simulink library "dspspect3"  (Simulink 6.0)
undefined symbols (not defined in the file or in its folder): D, magnitude
libraries: dspspect3 x5, dspparest3 x4, dspsigattribs x2, dspsigops x2, dspxfrm3 x1, dsparch4 x1, simulink x1
settings Model: RequirementInfo=9  CovMetricSettings=d  ForwardingTableString=||__slOldName__||dspspect3/Short-Time FFT||__slNewName__||dspspect3/Periodogram  Creator=don  LastModifiedBy=sconahan  ExtModeAutoUpdateStatusClock=off  ProdHWDeviceType=Specified

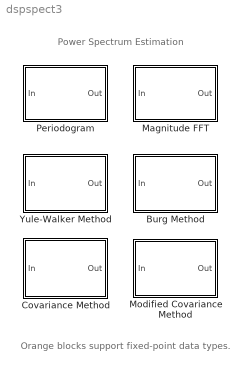
== system dspspect3 ==
  note: Power Spectrum Estimation
  note: Orange blocks support fixed-point data types.
  Burg Method : Subsystem  mask(Burg Method){inheritOrd=off, ord=6, inheritFFT=off, fftsize=256}
      mask prompts: inheritOrd "Inherit estimation order from input dimensions"; ord "Estimation order:"; inheritFFT "Inherit FFT length from estimation order"; fftsize "FFT length:"
      mask help: Parametric estimation of the AR spectrum using the Burg method.
      mask init:
      | [xe,x,y]=dspblkburgmeth2('icon');
      | dspblkburgmeth2('init');
      mask Help: web(dspbhelp);
      mask CallbackString: dspblkburgmeth2||dspblkburgmeth2|
      mask Display: text(-3,1.2,'Burg'); plot(-xe,0,xe,1.3,x,y)
  Covariance Method : Subsystem  mask(Covariance Method){ord=6, inheritFFT=off, fftsize=256}
      mask prompts: ord "Estimation order:"; inheritFFT "Inherit FFT length from estimation order"; fftsize "FFT length:"
      mask help: Parametric estimation of the AR spectrum using the covariance method.
      mask init:
      | [xe,x,y]=dspblkcovarmeth2('icon');
      | dspblkcovarmeth2('init');
      mask Help: web(dspbhelp);
      mask CallbackString: |dspblkcovarmeth2|
      mask Display: text(-3,1.2,'Cov AR'); plot(-xe,0,xe,1.3,x,y)
  Magnitude FFT : Subsystem  mask(Magnitude FFT){mag_or_magsq=Magnitude squared, fftLenInherit=off, fftsize=256}
      mask prompts: mag_or_magsq "Output:"; fftLenInherit "Inherit FFT length from input dimensions"; fftsize "FFT length:"
      mask help: Compute magnitude or magnitude-squared FFT of the input, with optional zero padding.
      mask init:
      | str=dspblkmagfft2('init');dspblkmagfft2('update');
      settings: CopyFcn=dspfixptcopycallback
      mask Help: web(dspbhelp);
      mask StyleString: popup(Magnitude squared|Magnitude),checkbox,edit
      mask CallbackString: |dspblkmagfft2;|
      mask Display: disp(str,'texmode','on');
  Modified Covariance Method : Subsystem  mask(Modified Covariance Method){ord=6, inheritFFT=off, fftsize=256}
      mask prompts: ord "Estimation order:"; inheritFFT "Inherit FFT length from estimation order"; fftsize "FFT length:"
      mask help: Parametric estimation of the AR spectrum using the modified covariance method.
      mask init:
      | [xe,x,y]=dspblkmodcovmeth2('icon');
      | dspblkmodcovmeth2('init');
      mask Help: web(dspbhelp);
      mask CallbackString: |dspblkmodcovmeth2|
      mask Display: text(-3,1.2,'MCov AR'); plot(-xe,0,xe,1.3,x,y)
  Periodogram : Subsystem  mask(Periodogram){wintype=Hamming, Rs=50, beta=5, winsamp=Symmetric, inheritFFT=off, fftsize=256, navg=4}
      mask prompts: wintype "Window type:"; Rs "Stopband attenuation in dB:"; winsamp "Window sampling:"; inheritFFT "Inherit FFT length from input dimensions"; fftsize "FFT length:"; navg "Number of spectral averages:"
      mask help: Nonparametric spectral estimation using the Periodogram method.
      mask init:
      | [x,y,xe]=dspblkshorttimefft2('icon');
      | dspblkshorttimefft2('init');
      mask Help: web(dspbhelp);
      mask StyleString: popup(Bartlett|Blackman|Boxcar|Chebyshev|Hamming|Hann|Hanning|Kaiser|Triang),edit,edit,popup(Symmetric|Periodic),checkbox,edit,edit
      mask CallbackString: dspblkshorttimefft2||||dspblkshorttimefft2||
      mask Display:
      | text(-3,1.15,'Periodogram');
      | plot((-xe),0,xe,1.3,x,y)
  Yule-Walker Method : Subsystem  mask(Yule-Walker Method){inheritOrd=off, ord=6, inheritFFT=off, fftsize=256}
      mask prompts: inheritOrd "Inherit estimation order from input dimensions"; ord "Estimation order:"; inheritFFT "Inherit FFT length from estimation order"; fftsize "FFT length:"
      mask help: Parametric estimation of the AR spectrum using the autocorrelation (LPC) method.
      mask init:
      | [xe,x,y]=dspblkyulewalkmeth2('icon');
      | dspblkyulewalkmeth2('init');
      mask Help: web(dspbhelp);
      mask CallbackString: dspblkyulewalkmeth2||dspblkyulewalkmeth2|
      mask Display: text(-3,1.2,'Yule AR'); plot(-xe,0,xe,1.3,x,y)

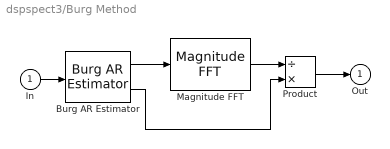
== system dspspect3/Burg Method ==
  In : Inport
  Burg AR Estimator : dspparest3/Burg AR Estimator  fcn=A  inheritOrder=off  ord=ord
  Magnitude FFT : dspspect3/Magnitude FFT  mag_or_magsq=Magnitude squared  fftLenInherit=off  fftsize=fftsize
  Product : Product  Inputs=/*  SaturateOnIntegerOverflow=on  InputSameDT=on
  Out : Outport  InitialOutput=0
  wires:
  In/1 -> Burg AR Estimator/1
  Burg AR Estimator/1 -> Magnitude FFT/1
  Magnitude FFT/1 -> Product/1
  Burg AR Estimator/2 -> Product/2
  Product/1 -> Out/1

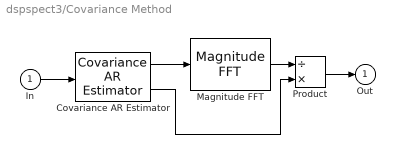
== system dspspect3/Covariance Method ==
  In : Inport
  Covariance AR Estimator : dspparest3/Covariance AR Estimator  P=ord
  Magnitude FFT : dspspect3/Magnitude FFT  mag_or_magsq=Magnitude squared  fftLenInherit=off  fftsize=fftsize
  Product : Product  Inputs=/*  SaturateOnIntegerOverflow=on  InputSameDT=on
  Out : Outport  InitialOutput=0
  wires:
  Magnitude FFT/1 -> Product/1
  Product/1 -> Out/1
  Covariance AR Estimator/1 -> Magnitude FFT/1
  Covariance AR Estimator/2 -> Product/2
  In/1 -> Covariance AR Estimator/1

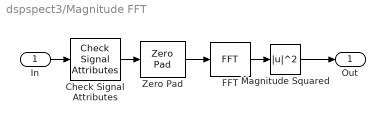
== system dspspect3/Magnitude FFT ==
  In : Inport
  Check Signal Attributes : dspsigattribs/Check Signal Attributes  SigAttribCheckMethod=Matches attributes exactly  Complexity=Ignore  Frame=Sample-based  DimsCheckMethod=Is...  Dimensions=Row vector (2-D)  DatatypeCheckMethod=Ignore  DatatypeGeneral=Boolean  DtypeFloatSpecific=Any floating-point  DtypeFixedSpecific=Any fixed-point  DtypeIntSpecific=Any integer  SampleMode=Ignore
  FFT : dspxfrm3/FFT  CompMethod=Table lookup  TableOpt=Speed  BitRevOrder=off  SkipNorm=on  roundingMode=Floor  overflowMode=off
  Magnitude Squared : Math  Operator=magnitude^2  ShowAdditionalParam=on  SaturateOnIntegerOverflow=on
  Zero Pad : dspsigops/Zero Pad  padSigAt=End  zpadAlong=Columns  padNumOutRowsSpecMethod=User-specified  numOutRows=fftsize  padNumOutColsSpecMethod=User-specified  numOutCols=1  trunc_flag=None
  Out : Outport
  wires:
  Magnitude Squared/1 -> Out/1
  In/1 -> Check Signal Attributes/1
  FFT/1 -> Magnitude Squared/1
  Zero Pad/1 -> FFT/1
  Check Signal Attributes/1 -> Zero Pad/1

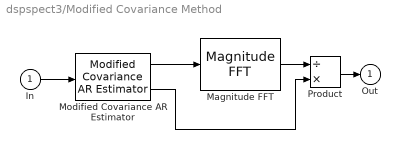
== system dspspect3/Modified Covariance Method ==
  In : Inport
  Magnitude FFT : dspspect3/Magnitude FFT  mag_or_magsq=Magnitude squared  fftLenInherit=off  fftsize=fftsize
  Modified Covariance AR Estimator : dspparest3/Modified Covariance AR Estimator  P=ord
  Product : Product  Inputs=/*  SaturateOnIntegerOverflow=on  InputSameDT=on
  Out : Outport  InitialOutput=0
  wires:
  In/1 -> Modified Covariance AR Estimator/1
  Modified Covariance AR Estimator/2 -> Product/2
  Modified Covariance AR Estimator/1 -> Magnitude FFT/1
  Product/1 -> Out/1
  Magnitude FFT/1 -> Product/1

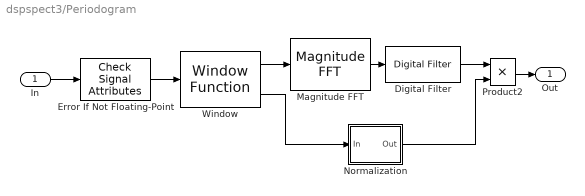
== system dspspect3/Periodogram ==
  In : Inport
  Digital Filter : dsparch4/Digital Filter  TypePopup=FIR (all zeros)  IIRFiltStruct=Direct form II transposed  AllPoleFiltStruct=Direct form  FIRFiltStruct=Direct form  CoeffSource=Specify via dialog  NumCoeffs=ones(navg,1)/navg  DenCoeffs=[1 0.1]  BiQuadCoeffs=[1 0.3 0.4 1 0.1 0.2]  LatticeCoeffs=[0.2 0.4]  denIgnore=on  FiltPerSampPopup=One filter per frame  IC=0  ICnum=0  ICden=0  roundingMode=Floor  overflowMode=off
  Error If Not Floating-Point : dspsigattribs/Check Signal Attributes  SigAttribCheckMethod=Does not match attributes exactly  Complexity=Ignore  Frame=Ignore  DimsCheckMethod=Ignore  Dimensions=1-D  DatatypeCheckMethod=Is...  DatatypeGeneral=Floating-point  DtypeFloatSpecific=Any floating-point  DtypeFixedSpecific=Any fixed-point  DtypeIntSpecific=Any integer  SampleMode=Ignore
  Magnitude FFT : dspspect3/Magnitude FFT  mag_or_magsq=Magnitude squared  fftLenInherit=off  fftsize=fftsize
  Normalization : Subsystem
  Product2 : Product  Inputs=**  SaturateOnIntegerOverflow=on  InputSameDT=on
  Window : dspsigops/Window Function  winmode=Generate and apply window  wintype=Hamming  sampmode=Continuous  samptime=1  N=64  Rs=Rs  beta=beta  winsamp=Symmetric  UserWindow=hamming  OptParams=off  UserParams={1.0}  dataType=double  wordLen=16  udDataType=sfix(16)  fracBitsMode=Best precision  numFracBits=15  roundingMode=Floor  overflowMode=off
      settings: additionalParams=on
  Out : Outport  InitialOutput=0
  wires:
  In/1 -> Error If Not Floating-Point/1
  Magnitude FFT/1 -> Digital Filter/1
  Window/1 -> Magnitude FFT/1
  Product2/1 -> Out/1
  Digital Filter/1 -> Product2/1
  Normalization/1(Out) -> Product2/2
  Window/2 -> Normalization/1(In)
  Error If Not Floating-Point/1 -> Window/1

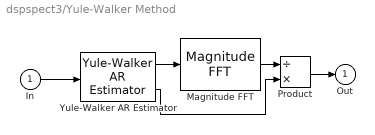
== system dspspect3/Yule-Walker Method ==
  In : Inport
  Magnitude FFT : dspspect3/Magnitude FFT  mag_or_magsq=Magnitude squared  fftLenInherit=off  fftsize=fftsize
  Product : Product  Inputs=/*  SaturateOnIntegerOverflow=on  InputSameDT=on
  Yule-Walker AR Estimator : dspparest3/Yule-Walker AR Estimator  ywArOutType=A  inheritOrder=off  ord=ord
  Out : Outport  InitialOutput=0
  wires:
  Product/1 -> Out/1
  Yule-Walker AR Estimator/1 -> Magnitude FFT/1
  Magnitude FFT/1 -> Product/1
  Yule-Walker AR Estimator/2 -> Product/2
  In/1 -> Yule-Walker AR Estimator/1

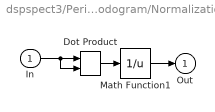
== system dspspect3/Periodogram/Normalization ==
  In : Inport
  Dot Product : simulink/Math Operations/Dot Product  OutDataType=sfix(16)  OutScaling=2^-10  DoSatur=off
  Math Function1 : Math  Operator=reciprocal  SaturateOnIntegerOverflow=on
  Out : Outport
  wires:
  Dot Product/1 -> Math Function1/1
  Math Function1/1 -> Out/1
  In/1 -> Dot Product/1, Dot Product/2
